simulink model "InitC22"  (R2020a)
settings: Solver=FixedStepAuto  StartTime=0.0  StopTime=10.0  FixedStep=1e-3  RelTol=1e-3  EnableMultiTasking=on
settings Model: ExtModeTrigDuration=5  Creator=WinnieTrandinh  LastModifiedBy=WinnieTrandinh
settings OptimizationCC: EnhancedBackFolding=on  PassReuseOutputArgsAs=Individual arguments  ZeroExternalMemoryAtStartup=off  ZeroInternalMemoryAtStartup=off  MaxStackSize=64  OptimizeBlockOrder=speed  DifferentSizesBufferReuse=on  OptimizationCustomize=off  EfficientTunableParamExpr=on
settings DebuggingCC: ParameterTunabilityLossMsg=error
settings HardwareCC: ProdBitPerPointer=32  ProdBitPerSizeT=32  ProdBitPerPtrDiffT=32  ProdLargestAtomicInteger=Long  ProdLargestAtomicFloat=Double  ProdWordSize=32  ProdHWDeviceType=ARM Compatible->ARM Cortex
settings SFSimCC: MATLABDynamicMemAlloc=off
settings RTWCC: SystemTargetFile=ert.tlc  HardwareBoard=NXP FRDM-K64F  TemplateMakefile=ert_default_tmf  Toolchain=GNU Tools for ARM Embedded Processors
settings CodeAppCC: ForceParamTrailComments=on  IgnoreCustomStorageClasses=off  OperatorAnnotations=on  SimulinkDataObjDesc=on  SFDataObjDesc=on  InsertBlockDesc=on

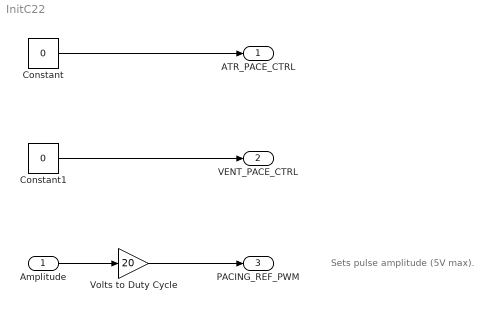
== system InitC22 ==
  note: Sets pulse amplitude (5V max).
  Amplitude : Inport
  Constant : Constant  Value=0
  Constant1 : Constant  Value=0
  Volts to Duty Cycle : Gain  Gain=20
  ATR_PACE_CTRL : Outport
  VENT_PACE_CTRL : Outport  Port=2
  PACING_REF_PWM : Outport  Port=3
  wires:
  Constant/1 -> ATR_PACE_CTRL/1
  Constant1/1 -> VENT_PACE_CTRL/1
  Amplitude/1 -> Volts to Duty Cycle/1
  Volts to Duty Cycle/1 -> PACING_REF_PWM/1
